simulink model "mvdc_disturbance_learning"  (R2018b)
settings: configuration reference "Active" (kept outside this file)
undefined symbols (not defined in the file): alg_mean_ax, alg_mean_ay, alg_quantile_ax_lower, alg_quantile_ax_upper, alg_quantile_ay_lower, alg_quantile_ay_upper
settings Model: DataDictionary=mvdc_disturbance_learning.sldd  Creator=wischnewski  LastModifiedBy=ge34qer

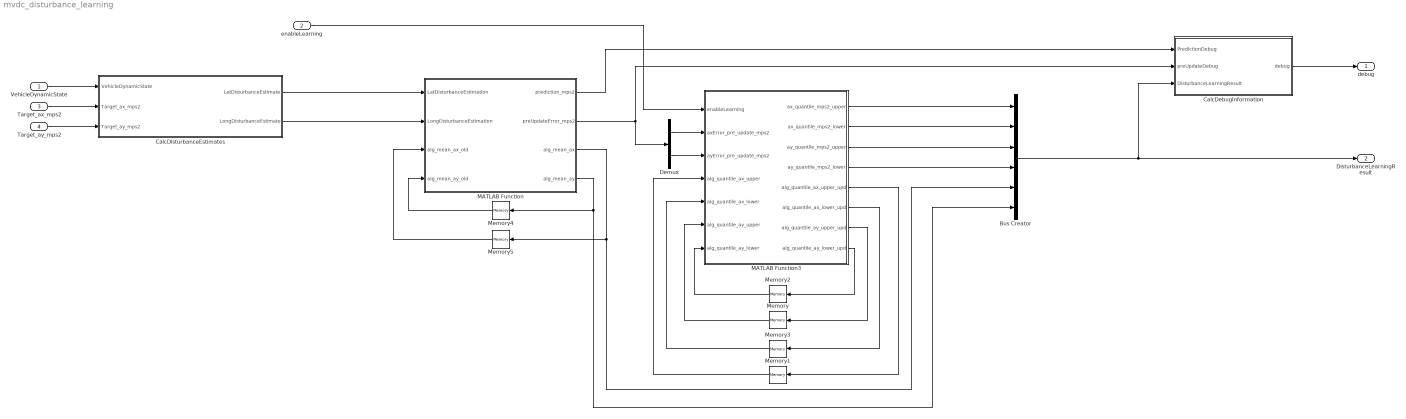
== system mvdc_disturbance_learning ==
  VehicleDynamicState : Inport  OutDataTypeStr=Bus: VehicleDynamicState
  enableLearning : Inport  Port=2  OutDataTypeStr=boolean
  Target_ax_mps2 : Inport  Port=3
  Target_ay_mps2 : Inport  Port=4
  Bus Creator : BusCreator  Inputs=6
  CalcDebugInformation : Subsystem
  CalcDisturbanceEstimates : Subsystem
  Demux : Demux  Outputs=2
  MATLAB Function : MATLAB Function  TreatAsAtomicUnit=on
  MATLAB Function3 : MATLAB Function  TreatAsAtomicUnit=on
  Memory : Memory  InitialCondition=alg_quantile_ay_upper
  Memory1 : Memory  InitialCondition=alg_quantile_ax_upper
  Memory2 : Memory  InitialCondition=alg_quantile_ay_lower
  Memory3 : Memory  InitialCondition=alg_quantile_ax_lower
  Memory4 : Memory  InitialCondition=alg_mean_ay
  Memory5 : Memory  InitialCondition=alg_mean_ax
  debug : Outport  OutDataTypeStr=Bus: mvdc_dist_learning_debug
  DisturbanceLearningResult : Outport  Port=2  OutDataTypeStr=Bus: DisturbanceLearningResult
  wires:
  CalcDebugInformation/1(debug) -> debug/1
  MATLAB Function/1(prediction_mps2) -> CalcDebugInformation/1(PredictionDebug)
  enableLearning/1 -> MATLAB Function3/1(enableLearning)
  Bus Creator/1 -> CalcDebugInformation/3(DisturbanceLearningResult), DisturbanceLearningResult/1
  MATLAB Function/2(preUpdateError_mps2) -> CalcDebugInformation/2(preUpdateDebug), Demux/1
  MATLAB Function3/2(ax_quantile_mps2_lower) -> Bus Creator/2
  MATLAB Function3/3(ay_quantile_mps2_upper) -> Bus Creator/3
  Demux/1 -> MATLAB Function3/2(axError_pre_update_mps2)
  Memory/1 -> MATLAB Function3/6(alg_quantile_ay_upper)
  Demux/2 -> MATLAB Function3/3(ayError_pre_update_mps2)
  MATLAB Function3/4(ay_quantile_mps2_lower) -> Bus Creator/4
  MATLAB Function3/1(ax_quantile_mps2_upper) -> Bus Creator/1
  Memory5/1 -> MATLAB Function/3(alg_mean_ax_old)
  MATLAB Function/4(alg_mean_ay) -> Bus Creator/6, Memory4/1
  MATLAB Function3/8(alg_quantile_ay_lower_upd) -> Memory2/1
  MATLAB Function/3(alg_mean_ax) -> Bus Creator/5, Memory5/1
  MATLAB Function3/6(alg_quantile_ax_lower_upd) -> Memory3/1
  MATLAB Function3/5(alg_quantile_ax_upper_upd) -> Memory1/1
  Memory3/1 -> MATLAB Function3/5(alg_quantile_ax_lower)
  Memory2/1 -> MATLAB Function3/7(alg_quantile_ay_lower)
  MATLAB Function3/7(alg_quantile_ay_upper_upd) -> Memory/1
  Memory4/1 -> MATLAB Function/4(alg_mean_ay_old)
  Memory1/1 -> MATLAB Function3/4(alg_quantile_ax_upper)
  CalcDisturbanceEstimates/2(LongDisturbanceEstimate) -> MATLAB Function/2(LongDisturbanceEstimation)
  VehicleDynamicState/1 -> CalcDisturbanceEstimates/1(VehicleDynamicState)
  Target_ax_mps2/1 -> CalcDisturbanceEstimates/2(Target_ax_mps2)
  Target_ay_mps2/1 -> CalcDisturbanceEstimates/3(Target_ay_mps2)
  CalcDisturbanceEstimates/1(LatDisturbanceEstimate) -> MATLAB Function/1(LatDisturbanceEstimation)

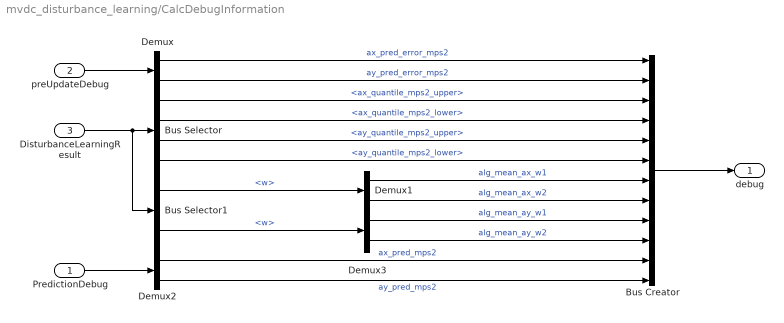
== system mvdc_disturbance_learning/CalcDebugInformation ==
  PredictionDebug : Inport
  preUpdateDebug : Inport  Port=2
  DisturbanceLearningResult : Inport  Port=3
  Bus Creator : BusCreator  Inputs=12
  Bus Selector : BusSelector  OutputSignals=ax_quantile_mps2_upper,ax_quantile_mps2_lower,ay_quantile_mps2_upper,ay_quantile_mps2_lower
  Bus Selector1 : BusSelector  OutputSignals=alg_mean_ax.w,alg_mean_ay.w
  Demux{,1..3} (4 alike) : Demux  Outputs=2
  debug : Outport
  wires:
  Bus Creator/1 -> debug/1
  Demux/1 -> Bus Creator/1  "ax_pred_error_mps2"
  Demux/2 -> Bus Creator/2  "ay_pred_error_mps2"
  DisturbanceLearningResult/1 -> Bus Selector1/1, Bus Selector/1
  Bus Selector/2 -> Bus Creator/4  "<ax_quantile_mps2_lower>"
  Bus Selector/1 -> Bus Creator/3  "<ax_quantile_mps2_upper>"
  Bus Selector/3 -> Bus Creator/5  "<ay_quantile_mps2_upper>"
  Bus Selector/4 -> Bus Creator/6  "<ay_quantile_mps2_lower>"
  Bus Selector1/1 -> Demux1/1  "<w>"
  Demux1/1 -> Bus Creator/7  "alg_mean_ax_w1"
  Demux1/2 -> Bus Creator/8  "alg_mean_ax_w2"
  Demux3/1 -> Bus Creator/9  "alg_mean_ay_w1"
  preUpdateDebug/1 -> Demux/1
  PredictionDebug/1 -> Demux2/1
  Demux2/1 -> Bus Creator/11  "ax_pred_mps2"
  Demux2/2 -> Bus Creator/12  "ay_pred_mps2"
  Bus Selector1/2 -> Demux3/1  "<w>"
  Demux3/2 -> Bus Creator/10  "alg_mean_ay_w2"

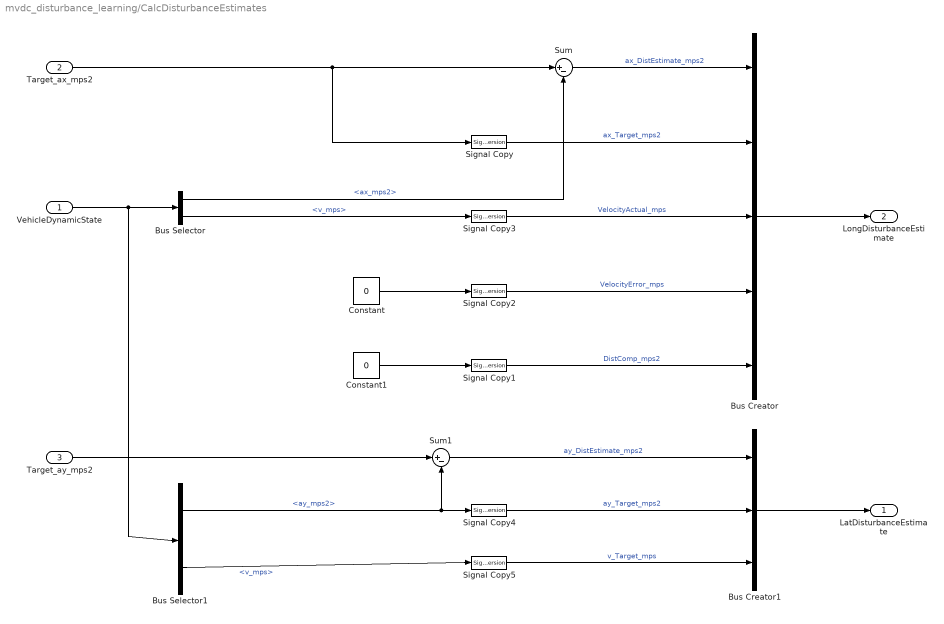
== system mvdc_disturbance_learning/CalcDisturbanceEstimates ==
  VehicleDynamicState : Inport  OutDataTypeStr=Bus: VehicleDynamicState
  Target_ax_mps2 : Inport  Port=2
  Target_ay_mps2 : Inport  Port=3
  Bus Creator : BusCreator  Inputs=5
  Bus Creator1 : BusCreator  Inputs=3
  Bus Selector : BusSelector  OutputSignals=ax_mps2,v_mps
  Bus Selector1 : BusSelector  OutputSignals=ay_mps2,v_mps
  Constant : Constant  Value=0
  Constant1 : Constant  Value=0
  Signal Copy{,1..5} (6 alike) : SignalConversion  OverrideOpt=off
  Sum : Sum  Inputs=|+-
  Sum1 : Sum  Inputs=|+-
  LatDisturbanceEstimate : Outport  OutDataTypeStr=Bus: LatDistEstimation
  LongDisturbanceEstimate : Outport  Port=2  OutDataTypeStr=Bus: LongDistEstimation
  wires:
  Sum/1 -> Bus Creator/1  "ax_DistEstimate_mps2"
  Bus Creator/1 -> LongDisturbanceEstimate/1
  Signal Copy/1 -> Bus Creator/2  "ax_Target_mps2"
  Signal Copy3/1 -> Bus Creator/3  "VelocityActual_mps"
  Signal Copy1/1 -> Bus Creator/5  "DistComp_mps2"
  Signal Copy2/1 -> Bus Creator/4  "VelocityError_mps"
  VehicleDynamicState/1 -> Bus Selector1/1, Bus Selector/1
  Bus Selector/2 -> Signal Copy3/1  "<v_mps>"
  Constant/1 -> Signal Copy2/1
  Constant1/1 -> Signal Copy1/1
  Target_ax_mps2/1 -> Signal Copy/1, Sum/1
  Bus Selector/1 -> Sum/2  "<ax_mps2>"
  Signal Copy4/1 -> Bus Creator1/2  "ay_Target_mps2"
  Signal Copy5/1 -> Bus Creator1/3  "v_Target_mps"
  Sum1/1 -> Bus Creator1/1  "ay_DistEstimate_mps2"
  Bus Creator1/1 -> LatDisturbanceEstimate/1
  Target_ay_mps2/1 -> Sum1/1
  Bus Selector1/1 -> Sum1/2, Signal Copy4/1  "<ay_mps2>"
  Bus Selector1/2 -> Signal Copy5/1  "<v_mps>"

== matlab function mvdc_disturbance_learning/MATLAB Function ==
  data: prediction_mps2 output size=2; LatDisturbanceEstimation input; LongDisturbanceEstimation input; preUpdateError_mps2 output size=2; alg_mean_ax output Bus: AlgMeanValueRegression; alg_mean_ay output Bus: AlgMeanValueRegression; alg_mean_ax_old input; alg_mean_ay_old input
function [prediction_mps2, preUpdateError_mps2, ...
    alg_mean_ax, alg_mean_ay]...
    = fcn(LatDisturbanceEstimation, LongDisturbanceEstimation, alg_mean_ax_old, alg_mean_ay_old)

% update mean prediction for longitudinal and lateral disturbance model
[ax_pre_update_mps2, alg_mean_ax] = learnDisturbanceMean(...
        [LongDisturbanceEstimation.ax_Target_mps2; ...
         LongDisturbanceEstimation.VelocityActual_mps^2],... 
         LongDisturbanceEstimation.ax_DistEstimate_mps2, alg_mean_ax_old); 
[ay_pre_update_mps2, alg_mean_ay] = learnDisturbanceMean(...
        [LatDisturbanceEstimation.ay_Target_mps2; 0],... 
         LatDisturbanceEstimation.ay_DistEstimate_mps2, alg_mean_ay_old); 
     
% calculate prediction error 
axError_pre_update_mps2 = LongDisturbanceEstimation.ax_DistEstimate_mps2 - ax_pre_update_mps2;
ayError_pre_update_mps2 = LatDisturbanceEstimation.ay_DistEstimate_mps2 - ay_pre_update_mps2; 

preUpdateError_mps2 = [axError_pre_update_mps2; ayError_pre_update_mps2]; 
prediction_mps2 = [ax_pre_update_mps2; ay_pre_update_mps2];

== matlab function mvdc_disturbance_learning/MATLAB Function3 ==
  data: enableLearning input boolean; ax_quantile_mps2_upper output double; ax_quantile_mps2_lower output double; ay_quantile_mps2_upper output double; ay_quantile_mps2_lower output double; alg_quantile_ax_upper_upd output Bus: AlgQuantileEstimation; alg_quantile_ax_lower_upd output Bus: AlgQuantileEstimation; alg_quantile_ay_upper_upd output Bus: AlgQuantileEstimation; axError_pre_update_mps2 input; ayError_pre_update_mps2 input; alg_quantile_ax_upper input Bus: AlgQuantileEstimation size=1; alg_quantile_ax_lower input Bus: AlgQuantileEstimation; alg_quantile_ay_upper input Bus: AlgQuantileEstimation size=1; alg_quantile_ay_lower_upd output Bus: AlgQuantileEstimation; alg_quantile_ay_lower input Bus: AlgQuantileEstimation
function [ax_quantile_mps2_upper, ax_quantile_mps2_lower, ay_quantile_mps2_upper, ay_quantile_mps2_lower,...
    alg_quantile_ax_upper_upd, alg_quantile_ax_lower_upd, alg_quantile_ay_upper_upd, alg_quantile_ay_lower_upd]...
    = fcn(enableLearning, axError_pre_update_mps2, ayError_pre_update_mps2, ...
    alg_quantile_ax_upper, alg_quantile_ax_lower, alg_quantile_ay_upper, alg_quantile_ay_lower)

if(enableLearning)
    % update quantile estimate for model error 
    alg_quantile_ax_upper_upd = learnDisturbanceQuantile(axError_pre_update_mps2, alg_quantile_ax_upper); 
    alg_quantile_ax_lower_upd = learnDisturbanceQuantile(axError_pre_update_mps2, alg_quantile_ax_lower); 
    alg_quantile_ay_upper_upd = learnDisturbanceQuantile(ayError_pre_update_mps2, alg_quantile_ay_upper); 
    alg_quantile_ay_lower_upd = learnDisturbanceQuantile(ayError_pre_update_mps2, alg_quantile_ay_lower); 
else
    alg_quantile_ax_upper_upd = alg_quantile_ax_upper; 
    alg_quantile_ax_lower_upd = alg_quantile_ax_lower; 
    alg_quantile_ay_upper_upd = alg_quantile_ay_upper; 
    alg_quantile_ay_lower_upd = alg_quantile_ay_lower; 
end

ax_quantile_mps2_upper = alg_quantile_ax_upper_upd.r_est; 
ax_quantile_mps2_lower = alg_quantile_ax_lower_upd.r_est; 
ay_quantile_mps2_upper = alg_quantile_ay_upper_upd.r_est;     
ay_quantile_mps2_lower = alg_quantile_ay_lower_upd.r_est;
